simulink model "cameraModel"  (R2023b)
settings: Solver=VariableStepAuto  StartTime=0.0  StopTime=106.138478597302  RelTol=1e-3
values from neighbouring files (symbols this model uses):
  cx = 640    [variablesInitialization.m]
  cy = 360    [variablesInitialization.m]
  fx = 1109    [variablesInitialization.m]
  fy = 1109    [variablesInitialization.m]
libraries: sim3dcameralib x4, dspvision x4, sim3dautolib x1, sim3dlib x1
settings Model: Creator=Hazem Abdelaziz  LastModifiedBy=Hazem Abdelaziz

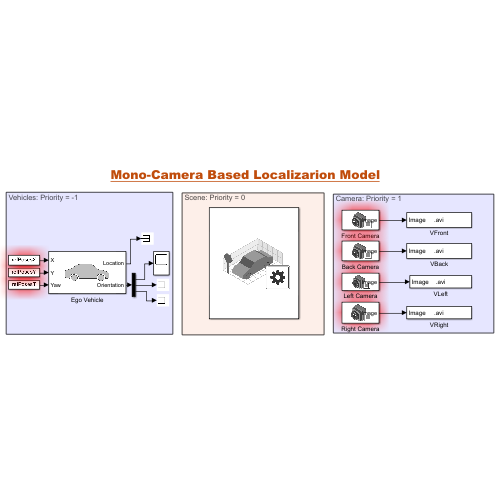
[thumbnail: Simulink's stored preview of the top-level diagram]
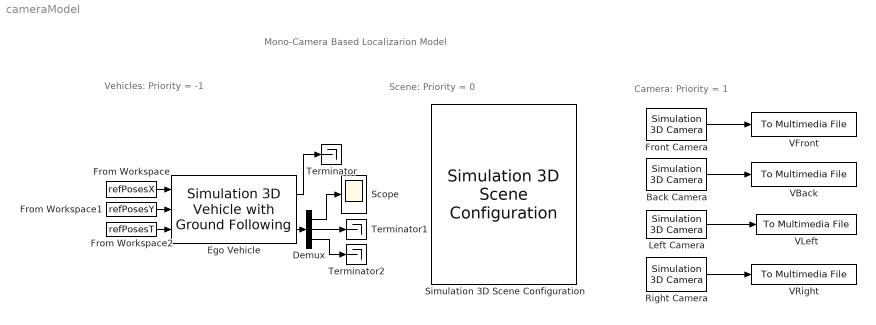
== system cameraModel ==
  note: Mono-Camera Based Localizarion Model
  note: Camera: Priority = 1
  note: Scene: Priority = 0
  note: Vehicles: Priority = -1
  Back Camera : sim3dcameralib/Simulation 3D Camera  Priority=1  sensorTag=Sim3dSensor2  sensorId=2  sensorName=Sim3dSensor2  vehTagList={'Scene Origin';'SimulinkVehicle1'}  vehTag=SimulinkVehicle1  mountLoc=Roof center  offsetFlag=on  tmountOffset=[-0.04, 0, 0]  extTmount=off  rmountOffset=[0, 0, 180]  extRmount=off  FocalLength=[fx, fy]  OpticalCenter=[cx, cy]  ImageSize=[720 1280]  RadialDistortion=[0, 0]  TangentialDistortion=[0, 0]  SensorSkew=0  DepthOutportEnabled=off  SemanticOutportEnabled=off  TransformOutportEnabled=off  SampleTime=-1  mountPoint=[-0.600000023841858 0 1.99000000953674]  mountOrientation=[0 0 -180]  aMode=3  ID=2
      settings: LibrarySourceBlock=drivingsim3d/Simulation 3D Camera
  Demux : Demux  Outputs=3
  Ego Vehicle : sim3dautolib/Simulation 3D Vehicle with Ground Following  Priority=-1  PassVehMesh=Sport utility vehicle  MeshPath=/MathWorksAutomotiveContent/Vehicles/Muscle/Meshes/SK_MuscleCar.SK_MuscleCar  TrackWidth=1.9  WheelBase=3  WheelRadius=0.35  VehColor=Blue  InitialPos=[-17.5108588917120, -11.1966058381202, 0]  InitialRot=[0, 0, 89.6327243900000]  ActorName=SimulinkVehicle1  SampleTime=-1  ActorType=SimulinkVehicle  ID=1  aMode=3  ActorTag=SimulinkVehicle1  CoordinateScheme=ISO  VehLightsControl=off  HeadlightColor=[ 1, 1, 1 ]  HighBeamIntensity=100000  LowBeamIntensity=60000  HighBeamConeAngle=70  LowBeamConeAngle=70  LeftHeadlightOrientation=[ 0, 0 ]  RightHeadlightOrientation=[ 0, 0 ]  BrakelightIntensity=500  ReverselightIntensity=500  SignallightIntensity=500  SignallightPeriod=1  SignalPulseWidth=50  TransformOutportEnabled=on
      settings: LibrarySourceBlock=drivingsim3d/Simulation 3D Vehicle with Ground Following
  From Workspace : FromWorkspace  VariableName=refPosesX
  From Workspace1 : FromWorkspace  VariableName=refPosesY
  From Workspace2 : FromWorkspace  VariableName=refPosesT
  Front Camera : sim3dcameralib/Simulation 3D Camera  Priority=1  sensorTag=Sim3dSensor1  sensorId=1  sensorName=Sim3dSensor1  vehTagList={'Scene Origin';'SimulinkVehicle1'}  vehTag=SimulinkVehicle1  mountLoc=Roof center  offsetFlag=off  tmountOffset=[0, 0.06, 0]  extTmount=off  rmountOffset=[0, 0, -0.2611]  extRmount=off  FocalLength=[fx, fy]  OpticalCenter=[cx, cy]  ImageSize=[720 1280]  RadialDistortion=[0, 0]  TangentialDistortion=[0, 0]  SensorSkew=0  DepthOutportEnabled=off  SemanticOutportEnabled=off  TransformOutportEnabled=off  SampleTime=-1  mountPoint=[-0.560000002384186 0 1.99000000953674]  mountOrientation=[0 0 0]  aMode=3  ID=1
      settings: LibrarySourceBlock=drivingsim3d/Simulation 3D Camera
  Left Camera : sim3dcameralib/Simulation 3D Camera  Priority=1  sensorTag=Sim3dSensor3  sensorId=3  sensorName=Sim3dSensor3  vehTagList={'Scene Origin';'SimulinkVehicle1'}  vehTag=SimulinkVehicle1  mountLoc=Roof center  offsetFlag=on  tmountOffset=[0, -0.06, 0]  extTmount=off  rmountOffset=[0, 0, 90]  extRmount=off  FocalLength=[fx, fy]  OpticalCenter=[cx, cy]  ImageSize=[720 1280]  RadialDistortion=[0, 0]  TangentialDistortion=[0, 0]  SensorSkew=0  DepthOutportEnabled=off  SemanticOutportEnabled=off  TransformOutportEnabled=off  SampleTime=-1  mountPoint=[-0.560000002384186 0.0599999986588955 1.99000000953674]  mountOrientation=[0 0 -90]  aMode=3  ID=3
      settings: LibrarySourceBlock=drivingsim3d/Simulation 3D Camera
  Right Camera : sim3dcameralib/Simulation 3D Camera  Priority=1  sensorTag=Sim3dSensor4  sensorId=4  sensorName=Sim3dSensor4  vehTagList={'Scene Origin';'SimulinkVehicle1'}  vehTag=SimulinkVehicle1  mountLoc=Roof center  offsetFlag=on  tmountOffset=[0, 0.06, 0]  extTmount=off  rmountOffset=[0, 0, -90]  extRmount=off  FocalLength=[fx, fy]  OpticalCenter=[cx, cy]  ImageSize=[720 1280]  RadialDistortion=[0, 0]  TangentialDistortion=[0, 0]  SensorSkew=0  DepthOutportEnabled=off  SemanticOutportEnabled=off  TransformOutportEnabled=off  SampleTime=-1  mountPoint=[-0.560000002384186 -0.0599999986588955 1.99000000953674]  mountOrientation=[0 0 90]  aMode=3  ID=4
      settings: LibrarySourceBlock=drivingsim3d/Simulation 3D Camera
  Scope : Scope
  Simulation 3D Scene Configuration : sim3dlib/Simulation 3D Scene Configuration  Priority=0  ProjectFormat=Default Scenes  SceneDesc=US city block  ProjectName=C:\Program Files\MATLAB\R2023b\toolbox\shared\sim3d_projects\automotive_project_windows\UE\WindowsNoEditor\VehicleSimulation.exe  ScenePath=/Game/Maps/HwStrght  EnableOpenDRIVE=off  vehTagList={'Custom';'Scene Origin';'SimulinkVehicle1'}  vehTag=SimulinkVehicle1  FreeCameraInitialTranslation=[0, 0, 0]  FreeCameraDefaultInitialTranslation=[-6, 0, 2]  FreeCameraInitialRotation=[0, 0, 0]  FreeCameraDefaultInitialRotation=[0, -15, 0]  OpVisEn=off  Ts=1/4.707  EnableWindow=on  EnableRemoteAccess=off  EnableWeather=off  SunAltitude=40.0  SunAzimuth=90  clouds=10  wind=1  fog=0  rain=0  EnableGeospatial=off  OriginHeight=200  OriginLatitude=40.744652  OriginLongitude=-73.988864  MapStyle=Aerial  AdditionalAssetIDs=[]  UseAdvancedSunSky=off  SolarTime=11  TimeZone=-5  Day=21  Month=9  Year=2022  UseDaylightSavingTime=on  DSTStartDay=10  DSTStartMonth=3  DSTEndDay=3  DSTEndMonth=11  DSTSwitchHour=2  sensorTag=MainCamera1  sensorId=1  sensorName=MainCamera1  mountLoc=Origin  offsetFlag=off  tmountOffset=[0, 0, 0]  rmountOffset=[0, 0, 0]  HorizontalResolution=1280  VerticalResolution=720  HorizontalFOV=60  mountPoint=[0 0 0]  mountOrientation=[0 0 0]  aMode=3  ID=1  GeoTrigger=Inactive
      settings: LibrarySourceBlock=drivingsim3d/Simulation 3D Scene Configuration
  Terminator : Terminator
  Terminator1 : Terminator
  Terminator2 : Terminator
  VBack : dspvision/To Multimedia File  outputFilename=.avi  streamSelection=Video only  videoCompressor=None (uncompressed)  audioCompressor=None (uncompressed)  imagePorts=One multidimensional signal  fileType=AVI  audioDatatype=Determine from input data type  fourcc=RGB  videoQuality=75  mj2000CompFactor=10
      settings: LibrarySourceBlock=visionsinks/To Multimedia File
  VFront : dspvision/To Multimedia File  outputFilename=.avi  streamSelection=Video only  videoCompressor=None (uncompressed)  audioCompressor=None (uncompressed)  imagePorts=One multidimensional signal  fileType=AVI  audioDatatype=Determine from input data type  fourcc=RGB  videoQuality=75  mj2000CompFactor=10
      settings: LibrarySourceBlock=visionsinks/To Multimedia File
  VLeft : dspvision/To Multimedia File  outputFilename=.avi  streamSelection=Video only  videoCompressor=None (uncompressed)  audioCompressor=None (uncompressed)  imagePorts=One multidimensional signal  fileType=AVI  audioDatatype=Determine from input data type  fourcc=RGB  videoQuality=75  mj2000CompFactor=10
      settings: LibrarySourceBlock=visionsinks/To Multimedia File
  VRight : dspvision/To Multimedia File  outputFilename=.avi  streamSelection=Video only  videoCompressor=None (uncompressed)  audioCompressor=None (uncompressed)  imagePorts=One multidimensional signal  fileType=AVI  audioDatatype=Determine from input data type  fourcc=RGB  videoQuality=75  mj2000CompFactor=10
      settings: LibrarySourceBlock=visionsinks/To Multimedia File
  wires:
  From Workspace2/1 -> Ego Vehicle/3
  Ego Vehicle/1 -> Terminator/1
  Ego Vehicle/2 -> Demux/1
  Demux/1 -> Scope/1
  Demux/2 -> Terminator1/1
  Demux/3 -> Terminator2/1
  Front Camera/1 -> VFront/1
  From Workspace/1 -> Ego Vehicle/1
  From Workspace1/1 -> Ego Vehicle/2
  Back Camera/1 -> VBack/1
  Right Camera/1 -> VRight/1
  Left Camera/1 -> VLeft/1
